simulink model "Microgrid_No_Attack"  (R2020b)
settings: Solver=VariableStepAuto  StartTime=0.0  StopTime=0.25  RelTol=1e-3
undefined symbols (not defined in the file): A_state_matrix_DG1, A_state_matrix_DG2, A_state_matrix_DG3, A_state_matrix_DG4, B_input_matrix_DG1, B_input_matrix_DG2, B_input_matrix_DG3, B_input_matrix_DG4, C_output_matrix_DG1, C_output_matrix_DG2, C_output_matrix_DG3, C_output_matrix_DG4, L_dot_DG1, L_dot_DG2, L_dot_DG3, L_dot_DG4
(part 1 of 2)
settings Model: Creator=RI  LastModifiedBy=andresintriagov
settings DataIOCC: SaveOutput=off  SaveTime=off  ReturnWorkspaceOutputs=off

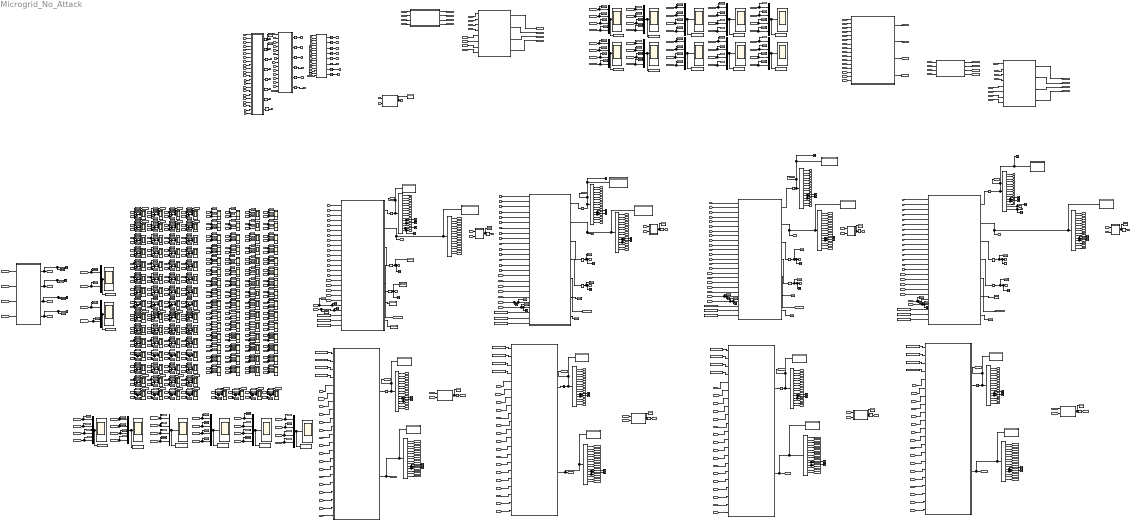
== system Microgrid_No_Attack ==
  " Vo_mag VCVSI1" : Scope
  " Vo_mag VCVSI3" : Scope
  Active Power VCVSI{1..4} (4 alike) : Scope
  Central Operation Values for VCVSI : Subsystem
  Constant1 : Constant  Value=A_state_matrix_DG1
  Constant10 : Constant  Value=A_state_matrix_DG3
  Constant11 : Constant  Value=B_input_matrix_DG3
  Constant12 : Constant  Value=C_output_matrix_DG3
  Constant13 : Constant  Value=A_state_matrix_DG4
  Constant14 : Constant  Value=B_input_matrix_DG4
  Constant15 : Constant  Value=C_output_matrix_DG4
  Constant16 : Constant  Value=L_dot_DG1
  Constant17 : Constant  Value=A_state_matrix_DG2
  Constant18 : Constant  Value=L_dot_DG2
  Constant19 : Constant  Value=B_input_matrix_DG2
  Constant2 : Constant  Value=B_input_matrix_DG1
  Constant20 : Constant  Value=C_output_matrix_DG2
  Constant21 : Constant  Value=A_state_matrix_DG3
  Constant22 : Constant  Value=L_dot_DG3
  Constant23 : Constant  Value=B_input_matrix_DG3
  Constant24 : Constant  Value=C_output_matrix_DG3
  Constant25 : Constant  Value=A_state_matrix_DG4
  Constant26 : Constant  Value=L_dot_DG4
  Constant27 : Constant  Value=B_input_matrix_DG4
  Constant28 : Constant  Value=C_output_matrix_DG4
  Constant3 : Constant  Value=C_output_matrix_DG1
  Constant4 : Constant  Value=A_state_matrix_DG1
  Constant5 : Constant  Value=B_input_matrix_DG1
  Constant6 : Constant  Value=C_output_matrix_DG1
  Constant7 : Constant  Value=A_state_matrix_DG2
  Constant8 : Constant  Value=B_input_matrix_DG2
  Constant9 : Constant  Value=C_output_matrix_DG2
  DG 1 Matrices : MATLAB Function  TreatAsAtomicUnit=on
  DG 2 Matrices : MATLAB Function  TreatAsAtomicUnit=on
  DG 3 Matrices : MATLAB Function  TreatAsAtomicUnit=on
  DG 4 Matrices : MATLAB Function  TreatAsAtomicUnit=on
  Demux{,1..15} (16 alike) : Demux  Outputs=15
  Display{,1..430,435,438..439,442} (435 alike) : Display
  Frequencies : MATLAB Function  TreatAsAtomicUnit=on
  Frequencies1 : MATLAB Function  TreatAsAtomicUnit=on
  Frequency VCVSI1 : Scope
  Frequency VCVSI3 : Scope
  Integrator{,1..3,65..67,73..75,77..84} (18 alike) : Integrator
  Integrator{4..7} (4 alike) : Integrator  InitialCondition=[0.1;0.1;0.1;0.1;0.1;0.1;0.1;0.1;0.1;0.1;0.1;0.1;0.1;0.1;0.1]
  L1_residual_error : Scope
  L2_residual_error : Scope
  LOAD : MATLAB Function  TreatAsAtomicUnit=on
  MATLAB Function1 : MATLAB Function  TreatAsAtomicUnit=on
  Mux{1..16} (16 alike) : Mux
  Mux17 : Mux  Inputs=2
  Mux18 : Mux  Inputs=2
  NET : MATLAB Function  TreatAsAtomicUnit=on
  OBSERVER DG 1 : MATLAB Function  TreatAsAtomicUnit=on
  OBSERVER DG 2 : MATLAB Function  TreatAsAtomicUnit=on
  OBSERVER DG 3 : MATLAB Function  TreatAsAtomicUnit=on
  OBSERVER DG 4 : MATLAB Function  TreatAsAtomicUnit=on
  Scope{,71..129} (60 alike) : Scope  NumInputPorts=2
  Scope{1..70,130..176,185..188} (121 alike) : Scope
  Sum{,1..63} (64 alike) : Sum  Inputs=|+-
  To Workspace1 : ToWorkspace  VariableName=vomagi  SaveFormat=Timeseries  SampleTime=-1
  To Workspace10 : ToWorkspace  VariableName=frequencies_hat  SaveFormat=Timeseries  SampleTime=-1
  To Workspace11 : ToWorkspace  VariableName=f_residual  SaveFormat=Timeseries  SampleTime=-1
  To Workspace12 : ToWorkspace  VariableName=L1_residual_error  SaveFormat=Timeseries  SampleTime=-1
  To Workspace13 : ToWorkspace  VariableName=L2_residual_error  SaveFormat=Timeseries  SampleTime=-1
  To Workspace15 : ToWorkspace  VariableName=x15_residual  SaveFormat=Timeseries  SampleTime=-1
  To Workspace16 : ToWorkspace  VariableName=x14_residual  SaveFormat=Timeseries  SampleTime=-1
  To Workspace17 : ToWorkspace  VariableName=x2_residual  SaveFormat=Timeseries  SampleTime=-1
  To Workspace18 : ToWorkspace  VariableName=x9_residual  SaveFormat=Timeseries  SampleTime=-1
  To Workspace2 : ToWorkspace  VariableName=vodi  SaveFormat=Timeseries  SampleTime=-1
  To Workspace20 : ToWorkspace  VariableName=x1_residual  SaveFormat=Timeseries  SampleTime=-1
  To Workspace3 : ToWorkspace  VariableName=active_power  SaveFormat=Timeseries  SampleTime=-1
  To Workspace4 : ToWorkspace  VariableName=reactive_power  SaveFormat=Timeseries  SampleTime=-1
  To Workspace5 : ToWorkspace  VariableName=vomagi_hat  SaveFormat=Timeseries  SampleTime=-1
  To Workspace6 : ToWorkspace  VariableName=vodi_hat  SaveFormat=Timeseries  SampleTime=-1
  To Workspace7 : ToWorkspace  VariableName=active_power_hat  SaveFormat=Timeseries  SampleTime=-1
  To Workspace8 : ToWorkspace  VariableName=frequencies  SaveFormat=Timeseries  SampleTime=-1
  To Workspace9 : ToWorkspace  VariableName=reactive_power_hat  SaveFormat=Timeseries  SampleTime=-1
  Transport Delay{1..24} (24 alike) : TransportDelay  DelayTime=0.0001
  VB : MATLAB Function  TreatAsAtomicUnit=on
  f_residual : Scope
  omega_1DG : MATLAB Function  TreatAsAtomicUnit=on
  omega_1DG_observer : MATLAB Function  TreatAsAtomicUnit=on
  omega_2DG : MATLAB Function  TreatAsAtomicUnit=on
  omega_2DG_observer : MATLAB Function  TreatAsAtomicUnit=on
  omega_3DG : MATLAB Function  TreatAsAtomicUnit=on
  omega_3DG_observer : MATLAB Function  TreatAsAtomicUnit=on
  omega_4DG : MATLAB Function  TreatAsAtomicUnit=on
  omega_4DG_observer : MATLAB Function  TreatAsAtomicUnit=on
  vod_voltages_VCVSI1 : Scope
  vod_voltages_VCVSI3 : Scope
  vomag : MATLAB Function  TreatAsAtomicUnit=on
  vomag1 : MATLAB Function  TreatAsAtomicUnit=on
  wcom : MATLAB Function  TreatAsAtomicUnit=on
  x14_residual : Scope
  x15_residual : Scope
  x1_residual : Scope
  x2_residual : Scope
  x9_residual : Scope
  wires:
  [x5_hat] -> Display216/1, Sum4/2
  Demux/15 -> Scope173/1, [x15]
  DG 2 Matrices/5(u_vector_DG2) -> [u_vector_DG2]
  [x14_1DG] -> omega_1DG/2(x14_1DG)
  [x17_hat] -> OBSERVER DG 2/8(x2_hat)
  Demux10/6 -> [x6_hat_1DG]
  Demux5/11 -> Scope54/1, [x41_3DG]
  [x60_hat] -> OBSERVER DG 4/21(x15_hat)
  Frequencies1/2(f2) -> [f2_hat]
  DG 4 Matrices/1(x_dot_DG4) -> Integrator3/1
  [x12] -> Display157/1, Scope81/1
  [x14_residual_DG4] -> Display399/1, Mux12/4
  [x9_hat] -> OBSERVER DG 1/15(x9_hat)
  [x9] -> vomag/1(x9)
  Sum49/1 -> Display360/1, Scope139/1
  Mux17/1 -> To Workspace12/1, L1_residual_error/1
  [x1_hat] -> OBSERVER DG 1/7(x1_hat)
  [P_matrix] -> DG 1 Matrices/16(P_matrix)
  [x14_residual_DG3] -> Display398/1, Mux12/3
  [x44] -> Display181/1, Scope113/1
  [x14_residual_DG1] -> Mux12/1, Display402/1
  [x32_hat] -> Display84/1, Scope101/2
  [x1] -> Central Operation Values for VCVSI/1(P_1DG)
  [Q_matrix] -> DG 4 Matrices/17(Q_matrix)
  [w4] -> Central Operation Values for VCVSI/12(w_4DG)
  [vbQ3] -> NET/12(vbQ3)
  Demux12/10 -> [x40_hat_3DG]
  Demux14/7 -> [x52_hat_4DG]
  [vbQ4] -> NET/14(vbQ4)
  [x47] -> DG 4 Matrices/2(x2)
  [x43] -> Display175/1, Scope112/1
  Demux11/15 -> [x30_hat_2DG]
  Demux9/12 -> Scope57/1, [x27_hat]
  [w1] -> Frequencies/1(w1)
  [x15] -> Sum14/1, Display245/1
  NET/4(xdot56) -> Integrator75/1
  [x55_hat] -> Display154/1, Scope124/2
  [x10_hat] -> OBSERVER DG 1/16(x10_hat)
  [x25] -> Sum29/1, Display274/1
  [x3_hat] -> Display210/1, Sum2/2
  Mux18/1 -> To Workspace13/1, L2_residual_error/1
  [x52] -> DG 4 Matrices/7(x7)
  [x37] -> DG 3 Matrices/7(x7)
  [x59] -> DG 4 Matrices/14(x14)
  Demux10/9 -> [x9_hat_1DG]
  Demux8/4 -> [x4_hat]
  Demux4/4 -> [x34]
  Demux3/10 -> [x25_2DG]
  Demux2/11 -> Scope33/1, [x26]
  [f1] -> Sum60/1, Display403/1
  Demux15/2 -> [x47_hat]
  Demux13/7 -> [x37_hat]
  [x1_residual_DG4] -> Display393/1, Mux15/4
  [Q_matrix] -> DG 1 Matrices/17(Q_matrix)
  Demux14/5 -> [x50_hat_4DG]
  Demux/4 -> [x4]
  VB/4(vbQ2) -> Transport Delay7/1
  [x14_residual_DG2] -> Display387/1, Mux12/2
  Demux14/13 -> [x58_hat_4DG]
  Frequencies1/3(f3) -> [f3_hat]
  [x60] -> Sum44/1, Display380/1
  Constant3/1 -> OBSERVER DG 1/3(C_output_matrix_DG1)
  [x27_hat] -> OBSERVER DG 2/18(x12_hat)
  [vbQ1] -> LOAD/10(vbQ1)
  [x56] -> Sum39/1, Display368/1
  Demux12/11 -> Scope29/1, [x41_hat_3DG]
  [L1_DG1] -> Display435/1, Mux17/1
  [u_vector_DG1] -> OBSERVER DG 1/6(u_vector_DG1)
  [f2] -> Sum61/1, Display406/1
  [y_DG1] -> OBSERVER DG 1/5(y_DG1)
  [x_hat_vector_DG1] -> MATLAB Function1/3(x_hat_vector_DG1)
  Sum9/1 -> Display232/1, Scope48/1
  Demux13/14 -> [x44_hat]
  [x33] -> DG 3 Matrices/3(x3)
  [x38] -> DG 3 Matrices/8(x8)
  [x58_hat] -> Display375/1, Sum41/2
  Transport Delay17/1 -> Display39/1, Scope18/1, [ioQ3]
  [x34_hat] -> OBSERVER DG 3/10(x4_hat)
  [x8] -> Sum7/1, Display223/1
  [x49_hat] -> OBSERVER DG 4/10(x4_hat)
  Demux8/2 -> [x2_hat]
  Demux13/8 -> [x38_hat]
  Demux5/12 -> Scope55/1, [x42_3DG]
  [x44_3DG] -> omega_3DG/2(x44_3DG)
  Integrator75/1 -> [x64]
  [x10_hat] -> Display150/1, Scope79/2
  [x15_hat] -> OBSERVER DG 1/21(x15_hat)
  [u_vector_DG3] -> OBSERVER DG 3/6(u_vector_DG3)
  [f4] -> Display26/1, Mux8/4
  [x2] -> Central Operation Values for VCVSI/5(Q_1DG)
  Demux8/12 -> Scope51/1, [x12_hat]
  [vbQ2] -> LOAD/12(vbQ2)
  [x1_hat] -> Display204/1, Sum/2
  [x59_hat] -> OBSERVER DG 4/20(x14_hat)
  Demux8/1 -> [x1_hat]
  [x52_hat] -> OBSERVER DG 4/13(x7_hat)
  Demux13/2 -> [x32_hat]
  [x2_residual_DG3] -> Mux13/3, Display394/1
  Transport Delay7/1 -> [vbQ2]
  [x9] -> Sum8/1, Display227/1
  Mux14/1 -> x9_residual/1, To Workspace18/1
  [x25_hat] -> vomag1/4(x25)
  [x41] -> Display163/1, Scope110/1
  Sum46/1 -> Display349/1, Scope166/1
  Demux5/3 -> [x33_3DG]
  Demux3/14 -> [x29_2DG]
  [u_vector_DG4] -> OBSERVER DG 4/6(u_vector_DG4)
  [x48_hat] -> OBSERVER DG 4/9(x3_hat)
  Demux10/5 -> [x5_hat_1DG]
  Transport Delay19/1 -> Display43/1, Scope23/1, [ioQ4]
  Constant22/1 -> OBSERVER DG 3/4(L_dot_DG3)
  [x39] -> Display31/1, Mux2/3
  [x25] -> Display148/1, Scope94/1
  [vbQ2] -> Display33/1, Scope14/1, DG 2 Matrices/22(vbQ2)
  Sum58/1 -> [x9_residual_DG3], Display321/1, Scope156/1
  [x13] -> Sum12/1, Display239/1
  Sum57/1 -> Display316/1, Scope155/1
  [x31] -> Central Operation Values for VCVSI/3(P_3DG)
  [x2_hat] -> Mux9/1, Display58/1
  VB/7(vbD4) -> Transport Delay10/1
  [x23_hat] -> Display269/1, Sum27/2
  Sum29/1 -> Display277/1, Scope133/1
  [vomag_1DG] -> Mux1/1, Display62/1
  LOAD/8(xdot66) -> Integrator80/1
  [f1_hat] -> Mux10/1, Display61/1
  MATLAB Function1/1(L1_DG1) -> Display427/1, Scope185/1, [L1_DG1]
  Demux3/3 -> [x18_2DG]
  Sum37/1 -> [x1_residual_DG4], Display342/1, Scope163/1
  Integrator3/1 -> [x_vector_DG4], Scope7/1, Display7/1, Demux6/1
  [x17] -> Display81/1, Scope86/1
  [x3_hat] -> Display92/1, Scope72/2
  LOAD/1(xdot59) -> Integrator78/1
  Demux9/5 -> [x20_hat]
  [wcom] -> LOAD/17(wcom)
  [x14_hat] -> Display194/1, Scope83/2
  Integrator6/1 -> [x_hat_vector_DG3], Display52/1, Demux13/1
  Demux6/11 -> Scope45/1, [x56]
  Demux6/3 -> [x48]
  [x54] -> DG 4 Matrices/9(x9)
  [x42] -> Display165/1, Scope111/1
  [x46] -> DG 4 Matrices/1(x1)
  [x1_hat] -> Display76/1, Scope/2
  Sum45/1 -> Display348/1, Scope165/1
  [f_residual_DG1] -> Mux16/1, Display415/1
  Sum38/1 -> [x2_residual_DG4], Display343/1, Scope164/1
  [x5] -> DG 1 Matrices/5(x5)
  [x39_hat] -> Display140/1, Scope108/2
  [x30_hat] -> Display291/1, Sum21/2
  [x21] -> Display121/1, Scope90/1
  [x4_hat] -> Display212/1, Sum3/2
  [x33_hat] -> Display96/1, Scope102/2
  [x9_hat] -> vomag1/1(x9)
  Demux7/5 -> [x50_4DG]
  Demux4/7 -> [x37]
  [x43] -> Sum34/1, Display329/1
  [x31] -> Display85/1, Scope100/1
  omega_3DG_observer/1(w3_observer) -> Transport Delay23/1, Display201/1
  [wcom] -> DG 3 Matrices/20(wcom)
  Central Operation Values for VCVSI/4(v_od_matrix) -> [v_od_matrix]
  Demux4/5 -> [x35]
  [x15] -> Display189/1, Scope84/1
  [x66] -> NET/6(x58)
  [x5_hat] -> Display116/1, Scope74/2
  [x53_hat] -> Display144/1, Scope122/2
  Demux11/10 -> [x25_hat_2DG]
  [x50_hat] -> Display351/1, Sum47/2
  Demux2/1 -> [x16]
  LOAD/4(xdot62) -> Integrator84/1
  [x46_hat] -> Mux7/4, Display71/1
  Sum23/1 -> Display259/1, Scope66/1
  Demux4/8 -> [x38]
  Constant9/1 -> DG 2 Matrices/25(C_output_matrix_DG2)
  [x_vector_DG1] -> MATLAB Function1/1(x_vector_DG1)
  Demux7/4 -> [x49_4DG]
  [x55_hat] -> Display365/1, Sum52/2
  [x45] -> Display185/1, Scope114/1
  Demux12/9 -> [x39_hat_3DG]
  Sum40/1 -> Display373/1, Scope144/1
  Sum13/1 -> [x14_residual_DG1], Display244/1, Scope59/1
  Demux4/2 -> [x32]
  Demux13/10 -> [x40_hat]
  [x17] -> DG 2 Matrices/2(x2)
  Demux10/12 -> Scope2/1, [x12_hat_1DG]
  [x30_hat] -> Display188/1, Scope99/2
  [x47_hat] -> OBSERVER DG 4/8(x2_hat)
  Demux12/4 -> [x34_hat_3DG]
  [x34_hat] -> Display104/1, Scope103/2
  [ioD2] -> VB/17(ioD2)
  Demux9/13 -> [x28_hat]
  [x52] -> Sum49/1, Display356/1
  [x26_hat] -> OBSERVER DG 2/17(x11_hat)
  [x31_hat] -> Mux7/3, Display69/1
  Transport Delay8/1 -> [vbD3]
  Sum39/1 -> Display372/1, Scope143/1
  [vbD1] -> NET/7(vbD1)
  [x62] -> NET/2(x54)
  [x5_hat] -> OBSERVER DG 1/11(x5_hat)
  omega_2DG/1(w2) -> Transport Delay21/1, Display45/1
  Demux/2 -> [x2]
  [vbQ1] -> NET/8(vbQ1)
  Demux10/10 -> [x10_hat_1DG]
  [x30] -> Sum21/1, Display290/1
  [f1_hat] -> Display404/1, Sum60/2
  Sum62/1 -> [f_residual_DG3], Display411/1, Scope171/1
  [x47] -> Mux4/4, Display30/1
  [x35] -> Display113/1, Scope104/1
  Sum33/1 -> Display328/1, Scope159/1
  [x9_residual_DG1] -> Mux14/1, Display385/1
  vomag1/3(vomag_3DG) -> [vomag_3DG_hat]
  [vbD3] -> LOAD/13(vbD3)
  [x54_hat] -> Display146/1, Scope123/2
  Mux7/1 -> Active Power VCVSI3/1, To Workspace7/1
  Sum44/1 -> [x15_residual_DG4], Display382/1, Scope147/1
  Demux1/10 -> [x10_1DG]
  Demux3/4 -> [x19_2DG]
  [x49_hat] -> Display106/1, Scope118/2
  [x13_hat] -> OBSERVER DG 1/19(x13_hat)
  [x28_hat] -> Display174/1, Scope97/2
  OBSERVER DG 2/1(x_hat_dot_DG2) -> Integrator5/1
  Demux1/2 -> [x2_1DG]
  Demux15/15 -> [x60_hat]
  [x4] -> Sum3/1, Display211/1
  [y_DG3] -> OBSERVER DG 3/5(y_DG3)
  [x32] -> DG 3 Matrices/2(x2)
  Sum31/1 -> [x2_residual_DG3], Display298/1, Scope149/1
  [L2_DG1] -> Display439/1, Mux18/1
  Demux2/13 -> [x28]
  [x36_hat] -> Display112/1, Scope105/2
  [x9_hat] -> Mux6/1, Display198/1
  [x10] -> Display147/1, Scope79/1
  LOAD/6(xdot64) -> Integrator82/1
  Constant28/1 -> OBSERVER DG 4/3(C_output_matrix_DG4)
  [x19_hat] -> Display257/1, Sum23/2
  [x1] -> Sum/1, Display203/1
  [x7] -> DG 1 Matrices/7(x7)
  [x16] -> Central Operation Values for VCVSI/2(P_2DG)
  [x9_hat] -> Display228/1, Sum8/2
  [vbD3] -> NET/11(vbD3)
  [v_od_matrix] -> DG 4 Matrices/19(v_od_matrix)
  [x46_hat] -> Display339/1, Sum37/2
  [x28_hat] -> Display285/1, Sum19/2
  [x22] -> DG 2 Matrices/7(x7)
  wcom/1(wcom) -> Display8/1, [wcom]
  [x61] -> VB/1(ilineD1)
  omega_1DG_observer/1(w1_observer) -> Transport Delay3/1, Display51/1
  [x72] -> VB/12(iloadQ3)
  Demux11/12 -> Scope26/1, [x27_hat_2DG]
  [x26_hat] -> Display160/1, Scope95/2
  Sum2/1 -> Display213/1, Scope37/1
  [x41_hat] -> OBSERVER DG 3/17(x11_hat)
  [x1_hat] -> Mux7/1, Display56/1
  [x18_hat] -> Display255/1, Sum22/2
  [x31_3DG] -> omega_3DG/1(x31_3DG)
  Integrator7/1 -> [x_hat_vector_DG4], Display54/1, Demux15/1
  DG 1 Matrices/1(x_dot_DG1) -> Integrator/1
  Constant10/1 -> DG 3 Matrices/23(A_state_matrix_DG3)
  Transport Delay6/1 -> [vbD2]
  [x29_hat] -> Display287/1, Sum20/2
  Demux/5 -> [x5]
  [x40] -> vomag/6(x40)
  Demux13/4 -> [x34_hat]
  [x23] -> DG 2 Matrices/8(x8)
  [ioD1] -> VB/15(ioD1)
  omega_1DG/1(w1) -> Transport Delay20/1, Display44/1
  [L1_DG4] -> Mux17/2, Display438/1
  [x44_hat_3DG] -> omega_3DG_observer/2(x44_hat_3DG)
  Demux8/9 -> [x9_hat]
  NET/5(xdot57) -> Integrator74/1
  omega_3DG/1(w3) -> Transport Delay1/1, Display46/1
  Transport Delay15/1 -> Display35/1, Scope13/1, [ioQ2]
  Demux10/13 -> [x13_hat_1DG]
  [x28] -> DG 2 Matrices/13(x13)
  DG 3 Matrices/3(ioD3) -> Transport Delay16/1
  [x59_4DG] -> omega_4DG/2(x59_4DG)
  Demux11/14 -> [x29_hat_2DG]
  [w1_observer] -> Frequencies1/1(w1)
  [x59_hat_4DG] -> omega_4DG_observer/2(x59_hat_4DG)
  Demux4/12 -> Scope40/1, [x42]
  Sum20/1 -> [x14_residual_DG2], Display289/1, Scope137/1
  Demux13/5 -> [x35_hat]
  [x24] -> vomag/3(x24)
  [x17] -> Display19/1, Mux4/2
  [x22_hat] -> Display267/1, Sum26/2
  [x6_hat] -> OBSERVER DG 1/12(x6_hat)
  [x2] -> DG 1 Matrices/2(x2)
  [x42_hat] -> Display326/1, Sum33/2
  Demux15/1 -> [x46_hat]
  [x60] -> DG 4 Matrices/15(x15)
  [x27] -> Sum18/1, Display280/1
  Demux14/9 -> [x54_hat_4DG]
  [x43] -> DG 3 Matrices/13(x13)
  DG 2 Matrices/1(x_dot_DG2) -> Integrator1/1
  Demux8/14 -> [x14_hat]
  [x20_hat] -> OBSERVER DG 2/11(x5_hat)
  Demux5/10 -> [x40_3DG]
  omega_4DG_observer/1(w4_observer) -> Transport Delay24/1, Display202/1
  Demux5/5 -> [x35_3DG]
  [x66] -> VB/6(ilineQ3)
  [x9_residual_DG4] -> Mux14/4, Display397/1
  [x52] -> Display141/1, Scope121/1
  [x10] -> vomag/2(x10)
  Demux4/13 -> [x43]
  VB/1(vbD1) -> Transport Delay4/1
  [L2_DG4] -> Mux18/2, Display442/1
  [x56_hat] -> Display168/1, Scope125/2
  [x48] -> DG 4 Matrices/3(x3)
  [x16] -> Display17/1, Mux3/2
  [x21] -> Sum25/1, Display262/1
  Demux1/13 -> [x13_1DG]
  [x51_hat] -> Display353/1, Sum48/2
  [x42] -> DG 3 Matrices/12(x12)
  [x54_hat] -> Display195/1, Mux6/4
  [vbD4] -> Display40/1, Scope21/1, DG 4 Matrices/21(vbD4)
  [wcom] -> DG 2 Matrices/20(wcom)
  [f_residual_DG4] -> Mux16/4, Display418/1
  [ioD4] -> VB/21(ioD4)
  Demux3/12 -> Scope50/1, [x27_2DG]
  [x12_hat] -> Display158/1, Scope81/2
  Integrator67/1 -> [x62]
  [x31] -> Sum30/1, Display293/1
  Sum18/1 -> Display283/1, Scope135/1
  [x11] -> Display155/1, Scope80/1
  [x16_hat] -> Display249/1, Sum15/2
  [x24_hat] -> Display130/1, Scope93/2
  [x57_hat] -> Display371/1, Sum40/2
  [x18] -> Display93/1, Scope87/1
  Integrator73/1 -> [x66]
  Integrator1/1 -> [x_vector_DG2], Scope5/1, Display5/1, Demux2/1
  [vomag_4DG] -> Display24/1, Mux1/4
  [vbD4] -> LOAD/15(vbD4)
  [x14] -> Sum13/1, Display241/1
  [x28] -> Sum19/1, Display284/1
  Demux7/13 -> [x58_4DG]
  Demux3/13 -> [x28_2DG]
  [x37_hat] -> Display136/1, Scope106/2
  [x7] -> Sum6/1, Display221/1
  [x4] -> Display99/1, Scope73/1
  Mux2/1 -> To Workspace2/1, vod_voltages_VCVSI3/1
  [x55] -> vomag/8(x55)
  VB/5(vbD3) -> Transport Delay8/1
  [x3] -> Sum2/1, Display209/1
  MATLAB Function1/4(L2_DG4) -> Display430/1, Scope188/1, [L2_DG4]
  Sum59/1 -> Display322/1, Scope157/1
  [x39_hat] -> vomag1/5(x39)
  Constant26/1 -> OBSERVER DG 4/4(L_dot_DG4)
  [x47_hat] -> Display90/1, Scope116/2
  Constant1/1 -> OBSERVER DG 1/1(A_state_matrix_DG1)
  [x53] -> DG 4 Matrices/8(x8)
  [x56_hat] -> Display369/1, Sum39/2
  Demux10/14 -> [x14_hat_1DG]
  NET/3(xdot55) -> Integrator65/1
  [vbD2] -> LOAD/11(vbD2)
  Transport Delay5/1 -> Display10/1, [vbQ1]
  [vomag_3DG_hat] -> Display64/1, Mux5/3
  Demux9/6 -> [x21_hat]
  [x50_hat] -> OBSERVER DG 4/11(x5_hat)
  [x39_hat] -> Display318/1, Sum58/2
  [x27_hat] -> Display281/1, Sum18/2
  NET/6(xdot58) -> Integrator73/1
  [x29] -> DG 2 Matrices/14(x14)
  Demux8/10 -> [x10_hat]
  Sum42/1 -> Display303/1, Scope150/1
  Integrator84/1 -> [x70]
  Frequencies/1(f1) -> [f1]
  Demux/13 -> [x13]
  [x53] -> Sum50/1, Display358/1
  [x39] -> Central Operation Values for VCVSI/15(v_od_3DG)
  [f3_hat] -> Display67/1, Mux10/3
  [x64] -> VB/4(ilineQ2)
  Demux12/15 -> [x45_hat_3DG]
  [x55] -> DG 4 Matrices/10(x10)
  Frequencies/4(f4) -> [f4]
  VB/2(vbQ1) -> Transport Delay5/1
  Integrator80/1 -> [x74]
  Demux1/5 -> [x5_1DG]
  [x24] -> DG 2 Matrices/9(x9)
  [x52_hat] -> Display142/1, Scope121/2
  [x59] -> Sum43/1, Display376/1
  Demux3/9 -> [x24_2DG]
  Demux2/2 -> [x17]
  Demux6/12 -> Scope46/1, [x57]
  [x9_residual_DG3] -> Display396/1, Mux14/3
  Demux13/13 -> [x43_hat]
  DG 4 Matrices/4(ioQ4) -> Transport Delay19/1
  [w4_observer] -> Frequencies1/4(w4)
  [x47] -> Display89/1, Scope116/1
  Demux7/7 -> [x52_4DG]
  [x20_hat] -> Display120/1, Scope89/2
  [x55_hat] -> vomag1/8(x55)
  [x46_hat] -> OBSERVER DG 4/7(x1_hat)
  [x11_hat] -> Display156/1, Scope80/2
  [x32_hat] -> Display72/1, Mux9/3
  [x50] -> DG 4 Matrices/5(x5)
  Demux4/9 -> [x39]
  Demux2/14 -> [x29]
  [x18] -> Sum22/1, Display254/1
  [vbD2] -> Display15/1, DG 2 Matrices/21(vbD2), Scope15/1
  OBSERVER DG 4/1(x_hat_dot_DG4) -> Integrator7/1
  Sum12/1 -> Display243/1, Scope58/1
  [x17_hat] -> Display251/1, Sum16/2
  Sum27/1 -> Display271/1, Scope131/1
  [x40] -> DG 3 Matrices/10(x10)
  [x48_hat] -> Display345/1, Sum45/2
  [f4] -> Sum63/1, Display412/1
  [x29] -> Sum20/1, Display286/1
  [x22] -> Display133/1, Scope91/1
  [x1_1DG] -> omega_1DG/1(x1_1DG)
  Demux14/15 -> [x60_hat_4DG]
  [x1] -> DG 1 Matrices/1(x1)
  Demux6/7 -> [x52]
  [x7] -> Display123/1, Scope76/1
  Transport Delay14/1 -> Display34/1, Scope12/1, [ioD2]
  Demux13/1 -> [x31_hat]
  [x1_residual_DG1] -> Mux15/1, Display388/1
  [x41_hat] -> Display164/1, Scope110/2
  [x74] -> VB/14(iloadQ4)
  [x56] -> Display167/1, Scope125/1
  [ioD3] -> VB/19(ioD3)
  Demux/3 -> [x3]
  [vomag_3DG] -> Display23/1, Mux1/3
  [x29] -> Display191/1, Scope98/1
  [x64] -> NET/4(x56)
  [x19_hat] -> OBSERVER DG 2/10(x4_hat)
  [x17_hat] -> Display59/1, Mux9/2
  [f3] -> Sum62/1, Display409/1
  Demux1/15 -> [x15_1DG]
  Sum60/1 -> [f_residual_DG1], Display405/1, Scope172/1
  Demux11/2 -> [x17_hat_2DG]
  DG 3 Matrices/1(x_dot_DG3) -> Integrator2/1
  Central Operation Values for VCVSI/1(P_matrix) -> [P_matrix]
  DG 2 Matrices/4(ioQ2) -> Transport Delay15/1
  [u_vector_DG2] -> OBSERVER DG 2/6(u_vector_DG2)
  [v_od_matrix] -> DG 3 Matrices/19(v_od_matrix)
  [x24_hat] -> Display273/1, Sum28/2
  Constant5/1 -> DG 1 Matrices/24(B_input_matrix_DG1)
  Demux7/10 -> [x55_4DG]
  Demux1/3 -> [x3_1DG]
  Sum30/1 -> [x1_residual_DG3], Display297/1, Scope148/1
  VB/3(vbD2) -> Transport Delay6/1
  [x16_hat_2DG] -> omega_2DG_observer/1(x16_hat_2DG)
  [x51] -> Sum48/1, Display352/1
  [vbQ4] -> Display41/1, Scope20/1, DG 4 Matrices/22(vbQ4)
  [x3] -> Display91/1, Scope72/1
  Demux11/3 -> [x18_hat_2DG]
  [x17] -> Central Operation Values for VCVSI/6(Q_2DG)
  Mux9/1 -> Active Power VCVSI4/1, To Workspace9/1
  Mux15/1 -> x1_residual/1, To Workspace20/1
  [x33] -> Display95/1, Scope102/1
  Sum28/1 -> [x9_residual_DG2], Display276/1, Scope132/1
  DG 3 Matrices/2(y_DG3) -> [y_DG3], Display2/1, Demux5/1
  [x2] -> Sum1/1, Display205/1
  [x63] -> NET/3(x55)
  [w3] -> Frequencies/3(w3)
  Transport Delay10/1 -> [vbD4]
  Sum51/1 -> [x9_residual_DG4], Display366/1, Scope141/1
  [wcom] -> DG 4 Matrices/20(wcom)
  [x21_hat] -> Display263/1, Sum25/2
  [x5] -> Sum4/1, Display215/1
  Sum56/1 -> Display315/1, Scope154/1
  [x58_hat] -> Display178/1, Scope127/2
  Constant14/1 -> DG 4 Matrices/24(B_input_matrix_DG4)
  [P_matrix] -> DG 2 Matrices/16(P_matrix)
  Mux10/1 -> Frequency VCVSI1/1, To Workspace10/1
  [x20] -> Sum24/1, Display260/1
  [x2] -> Display79/1, Scope71/1
  [Q_matrix] -> DG 3 Matrices/17(Q_matrix)
  [x49] -> Sum46/1, Display346/1
  [x5] -> Display115/1, Scope74/1
  [x12_hat] -> Display236/1, Sum11/2
  Constant25/1 -> OBSERVER DG 4/1(A_state_matrix_DG4)
  [x48] -> Sum45/1, Display344/1
  Frequencies/3(f3) -> [f3]
  [x8] -> DG 1 Matrices/8(x8)
  Demux8/7 -> [x7_hat]
  Mux8/1 -> Frequency VCVSI3/1, To Workspace8/1
  [w2] -> Central Operation Values for VCVSI/10(w_2DG)
  Demux2/15 -> [x30]
  [x24] -> Sum28/1, Display272/1
  [x29_2DG] -> omega_2DG/2(x29_2DG)
  [x6_hat] -> Display218/1, Sum5/2
  [x9] -> DG 1 Matrices/9(x9)
  Constant27/1 -> OBSERVER DG 4/2(B_input_matrix_DG4)
  Demux6/9 -> [x54]
  Sum7/1 -> Display226/1, Scope44/1
  [x4_hat] -> Display100/1, Scope73/2
  Demux/10 -> [x10]
  [f4_hat] -> Display68/1, Mux10/4
  [x52_hat] -> Display357/1, Sum49/2
  Demux7/1 -> [x46_4DG]
  [x58] -> DG 4 Matrices/13(x13)
  [x53_hat] -> Display359/1, Sum50/2
  [x50] -> Display107/1, Scope119/1
  DG 1 Matrices/3(ioD1) -> Transport Delay12/1
  [x31_hat] -> Display86/1, Scope100/2
  Demux5/14 -> [x44_3DG]
  [x1] -> Mux3/1, Display16/1
  [ioQ2] -> VB/18(ioQ2)
  [x38_hat] -> Display138/1, Scope107/2
  [x2_residual_DG4] -> Mux13/4, Display395/1
  Demux14/8 -> [x53_hat_4DG]
  Constant7/1 -> DG 2 Matrices/23(A_state_matrix_DG2)
  Demux12/13 -> [x43_hat_3DG]
  Sum36/1 -> [x15_residual_DG3], Display337/1, Scope162/1
  [x13_hat] -> Display172/1, Scope82/2
  [vomag_4DG_hat] -> Display65/1, Mux5/4
  DG 1 Matrices/5(u_vector_DG1) -> [u_vector_DG1]
  [x37_hat] -> OBSERVER DG 3/13(x7_hat)
  Demux2/7 -> [x22]
  [x49_hat] -> Display347/1, Sum46/2
  [vbD1] -> LOAD/9(vbD1)
  Central Operation Values for VCVSI/3(w_matrix) -> [w_matrix]
  [w4] -> Frequencies/4(w4)
  [x4] -> DG 1 Matrices/4(x4)
  Demux12/8 -> [x38_hat_3DG]
  [x23] -> Sum27/1, Display268/1
  [x31_hat] -> OBSERVER DG 3/7(x1_hat)
  [x36_hat] -> Display308/1, Sum55/2
  Sum43/1 -> [x14_residual_DG4], Display379/1, Scope146/1
  Mux6/1 -> To Workspace6/1, vod_voltages_VCVSI1/1
  [x11] -> DG 1 Matrices/11(x11)
  [x8] -> Display125/1, Scope77/1
  [vbQ4] -> LOAD/16(vbQ4)
  Integrator66/1 -> [x61]
  Demux15/6 -> [x51_hat]
  Demux14/2 -> [x47_hat_4DG]
  Demux11/9 -> [x24_hat_2DG]
  Demux14/11 -> Scope31/1, [x56_hat_4DG]
  [x24_hat] -> OBSERVER DG 2/15(x9_hat)
  Demux12/2 -> [x32_hat_3DG]
  [x39] -> Display139/1, Scope108/1
  Constant16/1 -> OBSERVER DG 1/4(L_dot_DG1)
  Constant6/1 -> DG 1 Matrices/25(C_output_matrix_DG1)
  [x9] -> Central Operation Values for VCVSI/13(v_od_1DG)
  [x24_hat] -> vomag1/3(x24)
  [x24] -> Central Operation Values for VCVSI/14(v_od_2DG)
  [x38] -> Sum57/1, Display313/1
  [x21_hat] -> Display122/1, Scope90/2
  [x27_hat] -> Display162/1, Scope96/2
  [x39] -> Sum58/1, Display317/1
  [x46] -> Sum37/1, Display338/1
  Demux14/12 -> Scope32/1, [x57_hat_4DG]
  [x29_hat] -> OBSERVER DG 2/20(x14_hat)
  Constant4/1 -> DG 1 Matrices/23(A_state_matrix_DG1)
  [x25_hat] -> OBSERVER DG 2/16(x10_hat)
  [x45_hat] -> OBSERVER DG 3/21(x15_hat)
  Demux9/3 -> [x18_hat]
  Transport Delay21/1 -> [w2]
  Demux5/7 -> [x37_3DG]
  Demux6/1 -> [x46]
  Demux1/11 -> [x11_1DG]
  Demux/6 -> [x6]
  [vbQ1] -> Display14/1, Scope11/1, DG 1 Matrices/22(vbQ1)
  [x59_hat] -> Display180/1, Scope128/2
  vomag1/4(vomag_4DG) -> [vomag_4DG_hat]
  Demux7/2 -> [x47_4DG]
  DG 2 Matrices/3(ioD2) -> Transport Delay14/1
  Demux10/1 -> [x1_hat_1DG]
  [x25_hat] -> Display149/1, Scope94/2
  [x56] -> DG 4 Matrices/11(x11)
  [x70] -> LOAD/4(x62)
  Sum15/1 -> Scope61/1, [x1_residual_DG2], Display252/1
  Transport Delay4/1 -> Display9/1, [vbD1]
  Demux5/6 -> [x36_3DG]
  Sum21/1 -> [x15_residual_DG2], Display292/1, Scope138/1
  [x31_hat_3DG] -> omega_3DG_observer/1(x31_hat_3DG)
  Transport Delay13/1 -> Display12/1, Scope9/1, [ioQ1]
  Central Operation Values for VCVSI/2(Q_matrix) -> [Q_matrix]
  Demux14/10 -> [x55_hat_4DG]
  [x29_hat_2DG] -> omega_2DG_observer/2(x29_hat_2DG)
  Demux8/8 -> [x8_hat]
  [x57_hat] -> OBSERVER DG 4/18(x12_hat)
  Demux7/12 -> Scope24/1, [x57_4DG]
  Demux2/12 -> Scope34/1, [x27]
  Demux1/9 -> [x9_1DG]
  [f_residual_DG2] -> Display416/1, Mux16/2
  [w2] -> Frequencies/2(w2)
  [x55_hat] -> OBSERVER DG 4/16(x10_hat)
  [x31_hat] -> Display294/1, Sum30/2
  [x_hat_vector_DG4] -> MATLAB Function1/4(x_hat_vector_DG4)
  [w_matrix] -> DG 3 Matrices/18(w_matrix)
  Sum4/1 -> Display219/1, Scope41/1
  omega_4DG/1(w4) -> Transport Delay2/1, Display47/1
  Demux13/6 -> [x36_hat]
  [x69] -> VB/9(iloadD2)
  [x46_hat] -> Display88/1, Scope115/2
  [f3_hat] -> Display410/1, Sum62/2
  [x29_hat] -> Display192/1, Scope98/2
  [x22] -> Sum26/1, Display266/1
  NET/1(xdot53) -> Integrator66/1
  Demux12/5 -> [x35_hat_3DG]
  Mux11/1 -> To Workspace15/1, x15_residual/1
  [x1_hat_1DG] -> omega_1DG_observer/1(x1_hat_1DG)
  [x40_hat] -> Display320/1, Sum59/2
  Demux7/11 -> Scope4/1, [x56_4DG]
  Demux5/13 -> [x43_3DG]
  [x32] -> Display29/1, Mux4/3
  Demux6/5 -> [x50]
  Demux9/2 -> [x17_hat]
  Sum19/1 -> Display288/1, Scope136/1
  [x18] -> DG 2 Matrices/3(x3)
  [ioQ1] -> VB/16(ioQ1)
  [x71] -> VB/11(iloadD3)
  Demux1/1 -> [x1_1DG]
  [f3] -> Display25/1, Mux8/3
  Integrator79/1 -> [x68]
  Demux/14 -> Scope174/1, [x14]
  [x14] -> DG 1 Matrices/14(x14)
  [x27] -> Display161/1, Scope96/1
  [x42_hat] -> Display166/1, Scope111/2
  VB/6(vbQ3) -> Transport Delay9/1
  Sum24/1 -> Display264/1, Scope67/1
  [x60_hat] -> Display381/1, Sum44/2
  [x56_hat] -> OBSERVER DG 4/17(x11_hat)
  [x47] -> Central Operation Values for VCVSI/8(Q_4DG)
  [x57] -> Display169/1, Scope126/1
  [x1_residual_DG2] -> Mux15/2, Display389/1
  Demux9/14 -> [x29_hat]
  [x3_hat] -> OBSERVER DG 1/9(x3_hat)
  Demux11/4 -> [x19_hat_2DG]
  [P_matrix] -> DG 3 Matrices/16(P_matrix)
  [x45_hat] -> Display186/1, Scope114/2
  Sum11/1 -> Display238/1, Scope53/1
  [x16] -> Sum15/1, Display248/1
  Constant8/1 -> DG 2 Matrices/24(B_input_matrix_DG2)
  [x19_hat] -> Display102/1, Scope88/2
  Demux/7 -> [x7]
  [x17_hat] -> Display82/1, Scope86/2
  [x19] -> DG 2 Matrices/4(x4)
  Demux10/4 -> [x4_hat_1DG]
  Sum/1 -> [x1_residual_DG1], Display207/1, Scope35/1
  Sum8/1 -> [x9_residual_DG1], Display231/1, Scope47/1
  Demux4/11 -> Scope39/1, [x41]
  [x35] -> Sum54/1, Display305/1
  [vbD1] -> Display13/1, Scope10/1, DG 1 Matrices/21(vbD1)
  Demux15/7 -> [x52_hat]
  [x19] -> Display101/1, Scope88/1
  [x43_hat] -> Display176/1, Scope112/2
  Sum6/1 -> Display225/1, Scope43/1
  [x63] -> VB/3(ilineD2)
  [x15_residual_DG3] -> Display390/1, Mux11/3
  [x16] -> Display77/1, Scope85/1
  [w_matrix] -> DG 2 Matrices/18(w_matrix)
  [x2] -> Mux4/1, Display18/1
  Demux15/4 -> [x49_hat]
  LOAD/5(xdot63) -> Integrator83/1
  [x14] -> Display193/1, Scope83/1
  Demux9/11 -> Scope56/1, [x26_hat]
  LOAD/2(xdot60) -> Integrator79/1
  [x6] -> Display117/1, Scope75/1
  Demux12/6 -> [x36_hat_3DG]
  [vbQ3] -> LOAD/14(vbQ3)
  [x45] -> DG 3 Matrices/15(x15)
  [x2_hat] -> Display80/1, Scope71/2
  Constant13/1 -> DG 4 Matrices/23(A_state_matrix_DG4)
  Demux6/2 -> [x47]
  Demux4/6 -> [x36]
  Sum63/1 -> [f_residual_DG4], Display414/1, Scope170/1
  [x61] -> NET/1(x53)
  Demux12/7 -> [x37_hat_3DG]
  vomag/3(vomag_3DG) -> [vomag_3DG]
  Integrator/1 -> [x_vector_DG1], Display4/1, Demux/1
  [x13] -> Display171/1, Scope82/1
  [x13_hat] -> Display240/1, Sum12/2
  [x1] -> wcom/1(x1)
  [x37] -> Sum56/1, Display311/1
  Demux7/9 -> [x54_4DG]
  Demux10/8 -> [x8_hat_1DG]
  [x70] -> VB/10(iloadQ2)
  [x39] -> DG 3 Matrices/9(x9)
  [x46] -> Central Operation Values for VCVSI/4(P_4DG)
  Demux2/4 -> [x19]
  Demux/8 -> [x8]
  [x54] -> Display145/1, Scope123/1
  Demux4/3 -> [x33]
  Transport Delay3/1 -> [w1_observer]
  [x45_hat] -> Display336/1, Sum36/2
  Demux11/13 -> [x28_hat_2DG]
  [x13] -> DG 1 Matrices/13(x13)
  Sum54/1 -> Display309/1, Scope152/1
  [ioQ3] -> VB/20(ioQ3)
  DG 3 Matrices/5(u_vector_DG3) -> [u_vector_DG3]
  [w3] -> Central Operation Values for VCVSI/11(w_3DG)
  [x25] -> vomag/4(x25)
  [x19] -> Sum23/1, Display256/1
  Demux8/6 -> [x6_hat]
  Sum52/1 -> Display367/1, Scope142/1
  Integrator82/1 -> [x72]
  Demux7/14 -> [x59_4DG]
  Integrator78/1 -> [x67]
  Transport Delay12/1 -> Display11/1, Scope8/1, [ioD1]
  Demux14/3 -> [x48_hat_4DG]
  [x3] -> DG 1 Matrices/3(x3)
  [x43_hat] -> OBSERVER DG 3/19(x13_hat)
  Constant24/1 -> OBSERVER DG 3/3(C_output_matrix_DG3)
  Transport Delay23/1 -> [w3_observer]
  [x9_residual_DG2] -> Display386/1, Mux14/2
  Sum41/1 -> Display378/1, Scope145/1
  [x30] -> DG 2 Matrices/15(x15)
  Demux3/11 -> Scope49/1, [x26_2DG]
  Frequencies/2(f2) -> [f2]
  [x60] -> Display183/1, Scope129/1
  Demux9/1 -> [x16_hat]
  [x37] -> Display135/1, Scope106/1
  [x35] -> DG 3 Matrices/5(x5)
  [x47_hat] -> Display341/1, Sum38/2
  Demux9/9 -> [x24_hat]
  Demux14/14 -> [x59_hat_4DG]
  [x38] -> Display137/1, Scope107/1
  DG 4 Matrices/5(u_vector_DG4) -> [u_vector_DG4]
  [x44_hat] -> Display182/1, Scope113/2
  LOAD/7(xdot65) -> Integrator81/1
  Transport Delay18/1 -> Display42/1, Scope22/1, [ioD4]
  Transport Delay1/1 -> [w3]
  Demux3/5 -> [x20_2DG]
  [x15_residual_DG1] -> Mux11/1, Display400/1
  [vbQ3] -> Display37/1, Scope16/1, DG 3 Matrices/22(vbQ3)
  Demux8/11 -> Scope3/1, [x11_hat]
  Demux7/6 -> [x51_4DG]
  [vbD3] -> Display36/1, Scope17/1, DG 3 Matrices/21(vbD3)
  [x2_residual_DG2] -> Display384/1, Mux13/2
  Integrator83/1 -> [x71]
  [x15_hat] -> Display246/1, Sum14/2
  [x34] -> DG 3 Matrices/4(x4)
  Integrator74/1 -> [x65]
  LOAD/3(xdot61) -> Integrator77/1
  Demux15/9 -> [x54_hat]
  [x51] -> DG 4 Matrices/6(x6)
  [x39] -> vomag/5(x39)
  [x33_hat] -> Display300/1, Sum42/2
  [w_matrix] -> DG 4 Matrices/18(w_matrix)
  [w_matrix] -> DG 1 Matrices/18(w_matrix)
  Sum25/1 -> Display265/1, Scope70/1
  Demux4/10 -> [x40]
  vomag/1(vomag_1DG) -> [vomag_1DG]
  [x22_hat] -> OBSERVER DG 2/13(x7_hat)
  Sum47/1 -> Display354/1, Scope167/1
  vomag1/2(vomag_2DG) -> [vomag_2DG_hat]
  Demux15/8 -> [x53_hat]
  Demux9/15 -> [x30_hat]
  Constant19/1 -> OBSERVER DG 2/2(B_input_matrix_DG2)
  Constant15/1 -> DG 4 Matrices/25(C_output_matrix_DG4)
  [x42_hat] -> OBSERVER DG 3/18(x12_hat)
  OBSERVER DG 1/2(y_hat_DG1) -> Display50/1, Demux10/1, [y_hat_DG1]
  Constant18/1 -> OBSERVER DG 2/4(L_dot_DG2)
  [x46_hat_4DG] -> omega_4DG_observer/1(x46_hat_4DG)
  [x58] -> Display177/1, Scope127/1
  Demux2/8 -> [x23]
  [x72] -> LOAD/6(x64)
  Transport Delay11/1 -> [vbQ4]
  [x47] -> Sum38/1, Display340/1
  Demux6/14 -> Scope176/1, [x59]
  [x15] -> DG 1 Matrices/15(x15)
  Demux6/15 -> Scope175/1, [x60]
  Demux5/15 -> [x45_3DG]
  [x44] -> DG 3 Matrices/14(x14)
  Demux/9 -> [x9]
  [x32] -> Sum31/1, Display295/1
  [x53_hat] -> OBSERVER DG 4/14(x8_hat)
  Demux12/12 -> Scope30/1, [x42_hat_3DG]
  [x23] -> Display131/1, Scope92/1
  [wcom] -> NET/15(wcom)
  [x59] -> Display179/1, Scope128/1
  [x68] -> LOAD/2(x60)
  Demux10/15 -> [x15_hat_1DG]
  Transport Delay20/1 -> [w1]
  [x40] -> Display151/1, Scope109/1
  [x25_hat] -> Display275/1, Sum29/2
  [x36] -> Sum55/1, Display307/1
  [x36_hat] -> OBSERVER DG 3/12(x6_hat)
  [x8_hat] -> OBSERVER DG 1/14(x8_hat)
  NET/2(xdot54) -> Integrator67/1
  Demux1/14 -> [x14_1DG]
  Demux8/15 -> [x15_hat]
  [x8_hat] -> Display126/1, Scope77/2
  Integrator2/1 -> Demux4/1, [x_vector_DG3], Scope6/1, Display6/1
  [x9] -> Mux2/1, Display70/1
  Demux15/12 -> Scope69/1, [x57_hat]
  [x11] -> Sum10/1, Display233/1
  [x48] -> Display97/1, Scope117/1
  [x14_hat_1DG] -> omega_1DG_observer/2(x14_hat_1DG)
  [x18_hat] -> OBSERVER DG 2/9(x3_hat)
  Constant20/1 -> OBSERVER DG 2/3(C_output_matrix_DG2)
  Demux3/1 -> [x16_2DG]
  OBSERVER DG 2/2(y_hat_DG2) -> Demux11/1, Display199/1, [y_hat_DG2]
  Sum17/1 -> Display282/1, Scope134/1
  [x7_hat] -> OBSERVER DG 1/13(x7_hat)
  [x40_hat] -> vomag1/6(x40)
  DG 4 Matrices/3(ioD4) -> Transport Delay18/1
  [x1_residual_DG3] -> Mux15/3, Display392/1
  [f2] -> Display22/1, Mux8/2
  Demux6/13 -> [x58]
  [x48_hat] -> Display98/1, Scope117/2
  [x26] -> Sum17/1, Display278/1
  Demux15/11 -> Scope68/1, [x56_hat]
  [x34] -> Sum53/1, Display301/1
  [x44_hat] -> Display332/1, Sum35/2
  Mux4/1 -> Active Power VCVSI2/1, To Workspace4/1
  [v_od_matrix] -> DG 2 Matrices/19(v_od_matrix)
  [vbQ2] -> NET/10(vbQ2)
  Demux/1 -> [x1]
  [x38_hat] -> Display314/1, Sum57/2
  Mux12/1 -> To Workspace16/1, x14_residual/1
  [x30_hat] -> OBSERVER DG 2/21(x15_hat)
  [x41_hat] -> Display324/1, Sum32/2
  [x33_hat] -> OBSERVER DG 3/9(x3_hat)
  Transport Delay9/1 -> [vbQ3]
  Demux9/8 -> [x23_hat]
  [x6] -> DG 1 Matrices/6(x6)
  Sum14/1 -> [x15_residual_DG1], Display247/1, Scope60/1
  [x55] -> Sum52/1, Display364/1
  Demux11/8 -> [x23_hat_2DG]
  Mux16/1 -> f_residual/1, To Workspace11/1
  [x12_hat] -> OBSERVER DG 1/18(x12_hat)
  Demux5/2 -> [x32_3DG]
  Demux6/10 -> [x55]
  [x20] -> Display119/1, Scope89/1
  [x51_hat] -> Display110/1, Scope120/2
  Sum26/1 -> Display270/1, Scope130/1
  [x10_hat] -> Display230/1, Sum9/2
  Demux13/3 -> [x33_hat]
  [x69] -> LOAD/3(x61)
  Demux8/13 -> [x13_hat]
  Integrator4/1 -> [x_hat_vector_DG1], Display48/1, Demux8/1
  [x37_hat] -> Display312/1, Sum56/2
  Demux11/1 -> [x16_hat_2DG]
  [x23_hat] -> Display132/1, Scope92/2
  Demux3/7 -> [x22_2DG]
  Demux12/1 -> [x31_hat_3DG]
  [x16_hat] -> OBSERVER DG 2/7(x1_hat)
  [x31] -> Mux3/3, Display27/1
  [f1] -> Mux8/1, Display21/1
  Constant23/1 -> OBSERVER DG 3/2(B_input_matrix_DG3)
  Demux10/11 -> Scope1/1, [x11_hat_1DG]
  omega_2DG_observer/1(w2_observer) -> Transport Delay22/1, Display200/1
  [x10_hat] -> vomag1/2(x10)
  [x71] -> LOAD/5(x63)
  Demux11/5 -> [x20_hat_2DG]
  [x65] -> VB/5(ilineD3)
  [x26_hat] -> Display279/1, Sum17/2
  Sum61/1 -> [f_residual_DG2], Display408/1, Scope169/1
  [x33] -> Sum42/1, Display299/1
  [x35_hat] -> Display114/1, Scope104/2
  [x55] -> Display153/1, Scope124/1
  Demux3/15 -> [x30_2DG]
  Constant2/1 -> OBSERVER DG 1/2(B_input_matrix_DG1)
  Mux5/1 -> To Workspace5/1, " Vo_mag VCVSI1"/1
  [w3_observer] -> Frequencies1/3(w3)
  [v_od_matrix] -> DG 1 Matrices/19(v_od_matrix)
  [x12] -> Sum11/1, Display235/1
  OBSERVER DG 3/1(x_hat_dot_DG3) -> Integrator6/1
  Demux11/11 -> Scope25/1, [x26_hat_2DG]
  [x57] -> DG 4 Matrices/12(x12)
  Sum34/1 -> Display333/1, Scope160/1
  OBSERVER DG 1/1(x_hat_dot_DG1) -> Integrator4/1
  [x32] -> Central Operation Values for VCVSI/7(Q_3DG)
  [x54] -> vomag/7(x54)
  [x40_hat] -> Display152/1, Scope109/2
  DG 4 Matrices/2(y_DG4) -> [y_DG4], Display3/1, Demux7/1
  [x51] -> Display109/1, Scope120/1
  [x32] -> Display83/1, Scope101/1
  [x46_4DG] -> omega_4DG/1(x46_4DG)
  [x16_hat] -> Display57/1, Mux7/2
  Demux4/15 -> [x45]
  Demux12/3 -> [x33_hat_3DG]
  Integrator77/1 -> [x69]
  [x62] -> VB/2(ilineQ1)
  Demux13/12 -> Scope63/1, [x42_hat]
  [x54_hat] -> vomag1/7(x54)
  [x17] -> Sum16/1, Display250/1
  Demux14/6 -> [x51_hat_4DG]
  [x49] -> DG 4 Matrices/4(x4)
  Demux14/4 -> [x49_hat_4DG]
  Demux15/14 -> [x59_hat]
  [x44] -> Sum35/1, Display331/1
  [x6] -> Sum5/1, Display217/1
  Demux1/12 -> [x12_1DG]
  Demux15/3 -> [x48_hat]
  [x24_hat] -> Display60/1, Mux6/2
  [x14] -> wcom/2(x14)
  [wcom] -> DG 1 Matrices/20(wcom)
  Sum22/1 -> Display258/1, Scope65/1
  [x15_residual_DG2] -> Display401/1, Mux11/2
  [x16_hat] -> Display78/1, Scope85/2
  [x7_hat] -> Display222/1, Sum6/2
  Demux13/9 -> [x39_hat]
  [x7_hat] -> Display124/1, Scope76/2
  [x9] -> Display127/1, Scope78/1
  [x12] -> DG 1 Matrices/12(x12)
  [x24] -> Display20/1, Mux2/2
  [f_residual_DG3] -> Display417/1, Mux16/3
  Demux13/11 -> Scope62/1, [x41_hat]
  [x40] -> Sum59/1, Display319/1
  [vbD2] -> NET/9(vbD2)
  Demux1/4 -> [x4_1DG]
  [x26] -> Display159/1, Scope95/1
  [x14_hat] -> OBSERVER DG 1/20(x14_hat)
  Frequencies1/4(f4) -> [f4_hat]
  Demux7/3 -> [x48_4DG]
  [x8_hat] -> Display224/1, Sum7/2
  [x15_hat] -> Display190/1, Scope84/2
  [x21] -> DG 2 Matrices/6(x6)
  vomag1/1(vomag_1DG) -> [vomag_1DG_hat]
  [x9_hat] -> Display128/1, Scope78/2
  [x50_hat] -> Display108/1, Scope119/2
  Demux9/10 -> [x25_hat]
  OBSERVER DG 4/2(y_hat_DG4) -> Display55/1, Demux14/1, [y_hat_DG4]
  Demux6/4 -> [x49]
  [x16_2DG] -> omega_2DG/1(x16_2DG)
  Demux10/7 -> [x7_hat_1DG]
  [x50] -> Sum47/1, Display350/1
  [x21_hat] -> OBSERVER DG 2/12(x6_hat)
  Sum35/1 -> [x14_residual_DG3], Display334/1, Scope161/1
  Integrator81/1 -> [x73]
  Demux8/3 -> [x3_hat]
  Demux5/4 -> [x34_3DG]
  Transport Delay2/1 -> [w4]
  [x10] -> Sum9/1, Display229/1
  [x36] -> Display111/1, Scope105/1
  [x24] -> Display129/1, Scope93/1
  Sum32/1 -> Display327/1, Scope158/1
  [P_matrix] -> DG 4 Matrices/16(P_matrix)
  [x65] -> NET/5(x57)
  Sum50/1 -> Display361/1, Scope140/1
  DG 3 Matrices/4(ioQ3) -> Transport Delay17/1
  Mux1/1 -> To Workspace1/1, " Vo_mag VCVSI3"/1
  [x25] -> DG 2 Matrices/10(x10)
  [x27] -> DG 2 Matrices/12(x12)
  Sum16/1 -> [x2_residual_DG2], Display253/1, Scope64/1
  Transport Delay24/1 -> [w4_observer]
  [x46] -> Mux3/4, Display28/1
  [x40_hat] -> OBSERVER DG 3/16(x10_hat)
  [x38_hat] -> OBSERVER DG 3/14(x8_hat)
  [x2_residual_DG1] -> Mux13/1, Display383/1
  [x26] -> DG 2 Matrices/11(x11)
  Demux5/8 -> [x38_3DG]
  [x51_hat] -> OBSERVER DG 4/12(x6_hat)
  Sum10/1 -> Display237/1, Scope52/1
  [x54] -> Sum51/1, Display362/1
  Demux1/8 -> [x8_1DG]
  Mux13/1 -> x2_residual/1, To Workspace17/1
  [x73] -> VB/13(iloadD4)
  [x41] -> DG 3 Matrices/11(x11)
  [f4_hat] -> Display413/1, Sum63/2
  Demux14/1 -> [x46_hat_4DG]
  [x57_hat] -> Display170/1, Scope126/2
  [x54_hat] -> Display363/1, Sum51/2
  [vomag_2DG_hat] -> Display197/1, Mux5/2
  Demux9/4 -> [x19_hat]
  OBSERVER DG 3/2(y_hat_DG3) -> Display53/1, Demux12/1, [y_hat_DG3]
  [x20_hat] -> Display261/1, Sum24/2
  Demux4/1 -> [x31]
  Demux1/6 -> [x6_1DG]
  Demux8/5 -> [x5_hat]
  Demux7/15 -> [x60_4DG]
  [vomag_2DG] -> Display66/1, Mux1/2
  Demux3/8 -> [x23_2DG]
  [x67] -> LOAD/1(x59)
  [ioQ4] -> VB/22(ioQ4)
  [vbD4] -> NET/13(vbD4)
  Demux15/5 -> [x50_hat]
  Sum53/1 -> Display304/1, Scope151/1
  [x6_hat] -> Display118/1, Scope75/2
  Demux/11 -> Scope27/1, [x11]
  Demux13/15 -> [x45_hat]
  Integrator5/1 -> [x_hat_vector_DG2], Display49/1, Demux9/1
  Demux1/7 -> [x7_1DG]
  Demux2/10 -> [x25]
  [x10] -> DG 1 Matrices/10(x10)
  [w2_observer] -> Frequencies1/2(w2)
  Constant21/1 -> OBSERVER DG 3/1(A_state_matrix_DG3)
  Transport Delay22/1 -> [w2_observer]
  [x54_hat] -> OBSERVER DG 4/15(x9_hat)
  [x28_hat] -> OBSERVER DG 2/19(x13_hat)
  [x47_hat] -> Mux9/4, Display73/1
  Demux2/3 -> [x18]
  Demux5/9 -> [x39_3DG]
  Demux10/3 -> [x3_hat_1DG]
  DG 1 Matrices/4(ioQ1) -> Transport Delay13/1
  [x43_hat] -> Display330/1, Sum34/2
  VB/8(vbQ4) -> Transport Delay11/1
  Sum48/1 -> Display355/1, Scope168/1
  Demux10/2 -> [x2_hat_1DG]
  [x42] -> Sum33/1, Display325/1
  MATLAB Function1/3(L1_DG4) -> Display429/1, Scope187/1, [L1_DG4]
  Sum1/1 -> [x2_residual_DG1], Display208/1, Scope36/1
  [y_DG2] -> OBSERVER DG 2/5(y_DG2)
  [x11_hat] -> OBSERVER DG 1/17(x11_hat)
  [x41] -> Sum32/1, Display323/1
  [x32_hat] -> Display296/1, Sum31/2
  [x49] -> Display105/1, Scope118/1
  [x67] -> VB/7(iloadD1)
  [x2_hat] -> Display206/1, Sum1/2
  [x14_hat] -> Display242/1, Sum13/2
  [x31] -> DG 3 Matrices/1(x1)
  DG 2 Matrices/2(y_DG2) -> [y_DG2], Display1/1, Demux3/1
  Sum5/1 -> Display220/1, Scope42/1
  vomag/4(vomag_4DG) -> [vomag_4DG]
  Constant17/1 -> OBSERVER DG 2/1(A_state_matrix_DG2)
  Sum55/1 -> Display310/1, Scope153/1
  [x34_hat] -> Display302/1, Sum53/2
  [x1] -> Scope/1, Display75/1
  [x22_hat] -> Display134/1, Scope91/2
  [x60_hat] -> Display184/1, Scope129/2
  [x68] -> VB/8(iloadQ1)
  vomag/2(vomag_2DG) -> [vomag_2DG]
  [w1] -> Central Operation Values for VCVSI/9(w_1DG)
  Demux11/7 -> [x22_hat_2DG]
  Mux3/1 -> Active Power VCVSI1/1, To Workspace3/1
  Demux6/6 -> [x51]
  MATLAB Function1/2(L2_DG1) -> Display428/1, Scope186/1, [L2_DG1]
  [x44_hat] -> OBSERVER DG 3/20(x14_hat)
  [x35_hat] -> Display306/1, Sum54/2
  Demux2/9 -> [x24]
  Demux4/14 -> [x44]
  [x53] -> Display143/1, Scope122/1
  [x_vector_DG4] -> MATLAB Function1/2(x_vector_DG4)
  Demux3/6 -> [x21_2DG]
  [x32_hat] -> OBSERVER DG 3/8(x2_hat)
  Demux11/6 -> [x21_hat_2DG]
  Demux6/8 -> [x53]
  Demux15/13 -> [x58_hat]
  [x39_hat] -> Display74/1, Mux6/3
  [x28] -> Display173/1, Scope97/1
  [x23_hat] -> OBSERVER DG 2/14(x8_hat)
  [x54] -> Display32/1, Mux2/4
  Demux9/7 -> [x22_hat]
  Demux5/1 -> [x31_3DG]
  [x20] -> DG 2 Matrices/5(x5)
  [x4_hat] -> OBSERVER DG 1/10(x4_hat)
  [x45] -> Sum36/1, Display335/1
  [x58_hat] -> OBSERVER DG 4/19(x13_hat)
  [x30] -> Display187/1, Scope99/1
  [x74] -> LOAD/8(x66)
  [f2_hat] -> Display407/1, Sum61/2
  [x73] -> LOAD/7(x65)
  Frequencies1/1(f1) -> [f1_hat]
  Sum3/1 -> Display214/1, Scope38/1
  [x2_hat] -> OBSERVER DG 1/8(x2_hat)
  Constant12/1 -> DG 3 Matrices/25(C_output_matrix_DG3)
  [x18_hat] -> Display94/1, Scope87/2
  Transport Delay16/1 -> Display38/1, Scope19/1, [ioD3]
  [x15_residual_DG4] -> Display391/1, Mux11/4
  Constant11/1 -> DG 3 Matrices/24(B_input_matrix_DG3)
  [Q_matrix] -> DG 2 Matrices/17(Q_matrix)
  Demux3/2 -> [x17_2DG]
  Demux2/5 -> [x20]
  Demux15/10 -> [x55_hat]
  Demux12/14 -> [x44_hat_3DG]
  [x16] -> DG 2 Matrices/1(x1)
  [x11_hat] -> Display234/1, Sum10/2
  Integrator65/1 -> [x63]
  [x34] -> Display103/1, Scope103/1
  [f2_hat] -> Display63/1, Mux10/2
  [x57] -> Sum40/1, Display370/1
  [x58] -> Sum41/1, Display374/1
  Demux7/8 -> [x53_4DG]
  [vomag_1DG_hat] -> Mux5/1, Display196/1
  [x46] -> Display87/1, Scope115/1
  DG 1 Matrices/2(y_DG1) -> [y_DG1], Demux1/1, Display/1
  Demux2/6 -> [x21]
  [y_DG4] -> OBSERVER DG 4/5(y_DG4)
  [x39_hat] -> OBSERVER DG 3/15(x9_hat)
  [x36] -> DG 3 Matrices/6(x6)
  [x59_hat] -> Display377/1, Sum43/2
  Demux/12 -> Scope28/1, [x12]
  [x35_hat] -> OBSERVER DG 3/11(x5_hat)
  [x54] -> Central Operation Values for VCVSI/16(v_od_4DG)
  DG 1 Matrices/7(vbq1) -> Display420/1
  DG 1 Matrices/6(vbd1) -> Display419/1
  DG 2 Matrices/6(vbd2) -> Display422/1
  DG 2 Matrices/7(vbq2) -> Display421/1
  DG 3 Matrices/6(vbd3) -> Display423/1
  DG 3 Matrices/7(vbq3) -> Display424/1
  DG 4 Matrices/6(vbd4) -> Display425/1
  DG 4 Matrices/7(vbq4) -> Display426/1

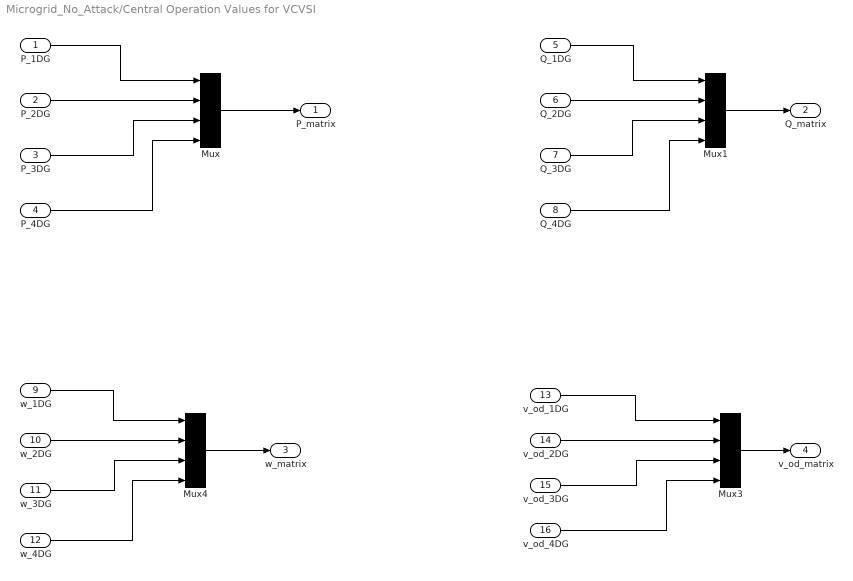
== system Microgrid_No_Attack/Central Operation Values for VCVSI ==
  P_1DG : Inport
  P_2DG : Inport  Port=2
  P_3DG : Inport  Port=3
  P_4DG : Inport  Port=4
  Q_1DG : Inport  Port=5
  Q_2DG : Inport  Port=6
  Q_3DG : Inport  Port=7
  Q_4DG : Inport  Port=8
  w_1DG : Inport  Port=9
  w_2DG : Inport  Port=10
  w_3DG : Inport  Port=11
  w_4DG : Inport  Port=12
  v_od_1DG : Inport  Port=13
  v_od_2DG : Inport  Port=14
  v_od_3DG : Inport  Port=15
  v_od_4DG : Inport  Port=16
  Mux{,1,3..4} (4 alike) : Mux
  P_matrix : Outport
  Q_matrix : Outport  Port=2
  w_matrix : Outport  Port=3
  v_od_matrix : Outport  Port=4
  wires:
  P_1DG/1 -> Mux/1
  P_2DG/1 -> Mux/2
  P_3DG/1 -> Mux/3
  Mux/1 -> P_matrix/1
  Q_2DG/1 -> Mux1/2
  Q_1DG/1 -> Mux1/1
  Q_3DG/1 -> Mux1/3
  Mux1/1 -> Q_matrix/1
  v_od_1DG/1 -> Mux3/1
  v_od_2DG/1 -> Mux3/2
  v_od_3DG/1 -> Mux3/3
  w_2DG/1 -> Mux4/2
  w_1DG/1 -> Mux4/1
  w_3DG/1 -> Mux4/3
  Mux4/1 -> w_matrix/1
  Mux3/1 -> v_od_matrix/1
  P_4DG/1 -> Mux/4
  Q_4DG/1 -> Mux1/4
  w_4DG/1 -> Mux4/4
  v_od_4DG/1 -> Mux3/4

== matlab function Microgrid_No_Attack/DG 4 Matrices ==
  data: x1 input; x_dot_DG4 output; x2 input; x3 input; x4 input; x5 input; x6 input; x7 input; x8 input; x9 input; x10 input; x11 input; x12 input; x13 input; x14 input; x15 input; y_DG4 output; P_matrix input; Q_matrix input; w_matrix input; v_od_matrix input; wcom input; vbD4 input; vbQ4 input; A_state_matrix_DG4 input; B_input_matrix_DG4 input; C_output_matrix_DG4 input; ioD4 output; ioQ4 output; u_vector_DG4 output; vbd4 output; vbq4 output
function [x_dot_DG4, y_DG4,ioD4,ioQ4, u_vector_DG4,vbd4,vbq4] = Matrices_SSM_DG4(x1,x2,x3,x4,x5,x6,x7,x8,x9,x10,x11,x12,x13,x14,x15,P_matrix, Q_matrix, w_matrix, v_od_matrix,wcom,vbD4,vbQ4,A_state_matrix_DG4,B_input_matrix_DG4,C_output_matrix_DG4)



Cf=50e-6;Lf=1.35e-3;rLf=.1;
Lc=.35e-3;rLc=.03;
wc=31.41;
mp1=9.4e-5;mp2=mp1;mp3=12.5e-5;mp4=mp3;


nq1=1.3e-3;nq2=nq1;nq3=1.5e-3;nq4=nq3;


Kpv1=.1;Kiv1=420;Kpv2=Kpv1;Kiv2=Kiv1;
Kpc1=15;Kic1=20*10^3;Kpc2=Kpc1;Kic2=Kic1;


Kpv3=.05;Kiv3=390;Kpv4=Kpv3;Kiv4=Kiv3;
Kpc3=10.5;Kic3=16*10^3;Kpc4=Kpc3;Kic4=Kic3;


F=.75;

wb=2*pi*50;

A_matrix= [0 0 0 0; 1 0 0 0; 1 0 0 0; 1 0 0 0]; %associated adjacency matrix
g_pinning_gain= [1;0;0;0]; %pinning gain vector
w_ref= 2*pi*50;
v_ref= 1;
c_f_2DG= 30;
c_v_2DG= 30;

m_P_1DG= 9.4*10^-5;
m_P_2DG= 9.4*10^-5;
m_P_3DG= 12.5*10^-5;
m_P_4DG= 12.5*10^-5;
n_Q_1DG= 1.3*10^-3;
n_Q_2DG= 1.3*10^-3; 
n_Q_3DG= 1.5*10^-3; 
n_Q_4DG= 1.5*10^-3; 

m_P_matrix= [m_P_1DG; m_P_2DG; m_P_3DG; m_P_4DG];
n_Q_matrix= [n_Q_1DG; n_Q_2DG; n_Q_3DG; n_Q_4DG];

vbd4=cos(x13)*vbD4+sin(x13)*vbQ4;vbq4=-sin(x13)*vbD4+cos(x13)*vbQ4;



%% Extracting several terms for x dot 14

%Obtaining a2_14 (term that is multiplied by x2 in x dot 14) (Active Power)



%Obtaining wj_input (cf*sum_aij*wj)

wj_input= 0;

for i=4
    for j= 1:4
        wj_input= (A_matrix(i,j)*w_matrix(j)) + wj_input;
    end
end

wj_input= wj_input*c_f_2DG;



%Obtaining wref_input (cf*gi*wref)


wref_input= c_f_2DG*g_pinning_gain(i)*w_ref;



%Obtaining Pj_input (cf*sum_aij*Pj)

Pj_input= 0;

for i= 4
    for j= 1:4
        Pj_input= (A_matrix(i,j)*m_P_matrix(j)*P_matrix(j)) + Pj_input;
    end
end

Pj_input= Pj_input*c_f_2DG;


        
%% Extracting several terms for x dot 15





%Obtaining vodj_input (cv*sum_aij*vodj)

vodj_input= 0;

for i= 4
    for j= 1:4
        vodj_input= (A_matrix(i,j)*v_od_matrix(j)) + vodj_input;
    end
end

vodj_input= c_v_2DG*vodj_input;


%Obtaining vref_input (cv*gi*vref)

vref_input= c_v_2DG*g_pinning_gain(i)*v_ref;


%Obtaining Qj_input (cv*sum_aij*Qj)

Qj_input= 0;

for i= 4
    for j= 1:4
        Qj_input= (A_matrix(i,j)*n_Q_matrix(j)*Q_matrix(j)) + Qj_input;
    end
end

Qj_input= c_v_2DG*Qj_input;




%% A matrix calculation

%A has 15 rows 15 columns

% x_vector=[alpha_i, P_i, Q_i, fi_d_i, fi_q_i,gamma_d_i,gamma_q_i, il_d_i, il_q_i, vo_d_i, vo_q_i,io_d_i,io_q_i,wni,Vni];


%% B Matrix Calculation 

%B has 15 rows 9 columns

u_vector_DG4= [wcom;vbd4;vbq4;wj_input;wref_input;Pj_input;vodj_input;vref_input;Qj_input];



%% C matrix calculation

% y=[wi; vodi; Pi; Qi;]

%C has 4 rows 15 columns


%% Non linear function (f) 15x1 

f_nonlinear_function=[
(wc*x9*x11) + (wc*x10*x12);
(-wc*x9*x12) + (wc*x10*x11);
0;
0;
0;
0;
(x14*x8) - (mp4*x1*x8);
(-x14*x7) + (mp4*x1*x7);
(x14*x10) - (mp4*x1*x10);
(-x14*x9) + (mp4*x1*x9);
(x14*x12) - (mp4*x1*x12);
(-x14*x11) + (mp4*x1*x11);
0;
0;
0;
];


%% x vector

x_vector_DG4= [x1;x2;x3;x4;x5;x6;x7;x8;x9;x10;x11;x12;x13;x14;x15];
%% xdot
x_dot_DG4= A_state_matrix_DG4*x_vector_DG4 + f_nonlinear_function + B_input_matrix_DG4*u_vector_DG4

y_DG4= C_output_matrix_DG4*x_vector_DG4


ioD4=cos(x13)*x11-sin(x13)*x12;
ioQ4=sin(x13)*x11+cos(x13)*x12;

== matlab function Microgrid_No_Attack/wcom ==
  data: x1 input; wcom output; x14 input
function wcom  = fcn(x1,x14)
mp1=9.4e-5;
wcom= x14 - mp1*x1
